simulink model "switching_deadtime_motor_model"  (R2023b)
settings: Solver=FixedStepDiscrete  StartTime=0.0  StopTime=0.002  FixedStep=ss_cfg.model_fixed_step_s  RelTol=1e-3
values from neighbouring files (symbols this model uses):
  phase = mod(t / T_pwm, 1.0)    [plot_phase_a_deadtime_comparison.m]    (also in run_mcu_sampling_window_study.m; run_rl_sampling_impact_study.m; run_rotating_rl_sampling_study.m; run_triangle_carrier_study.m)
  ss_cfg = local_parse_inputs(ss_cfg, varargin{:})    [run_switching_deadtime_motor_smoke_test.m]
libraries: simulink x2, spsDCVoltageSourceLib x1, motor_control_lib x1, spsPermanentMagnetSynchronousMachineLib x1, spsUniversalBridgeLib x1, spspowerguiLib x1
settings Model: DataDictionary=motor_control_interface.sldd  Creator=user  LastModifiedBy=user

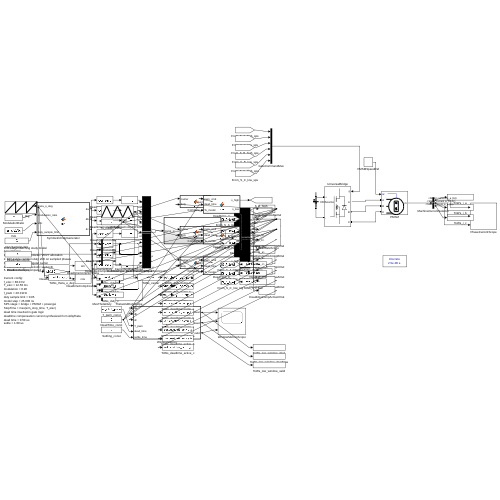
[thumbnail: Simulink's stored preview of the top-level diagram]
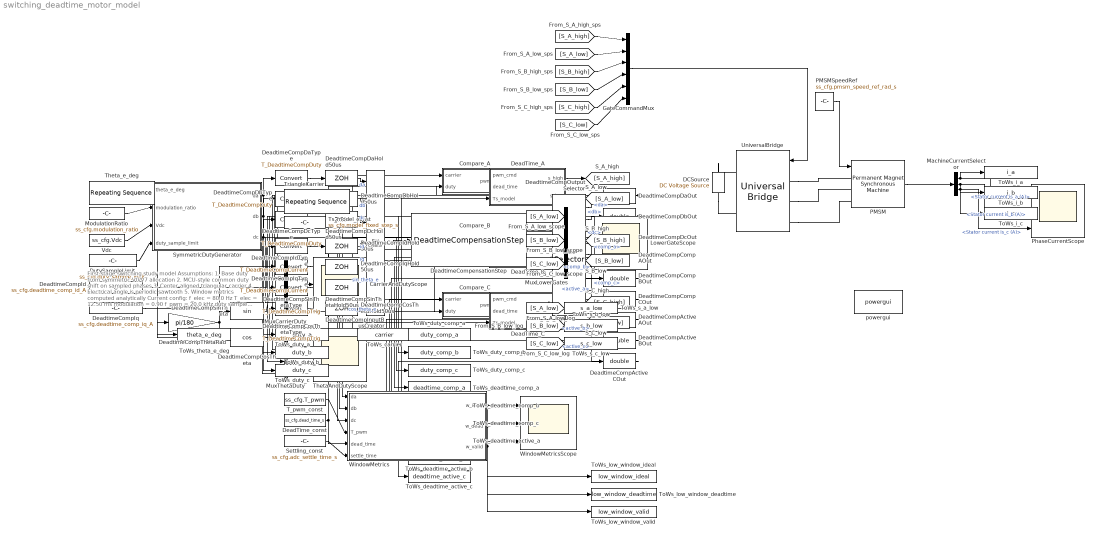
== system switching_deadtime_motor_model ==
  note: First-stage switching study model
      | Assumptions:
      | 1. Base duty from symmetric V0/V7 allocation
      | 2. MCU-style common duty shift on sampled phases
      | 3. Center-aligned triangular carrier
      | 4. Electrical angle is periodic sawtooth
      | 5. Window metrics computed analytically
      |
      | Current config:
      | f_elec = 80.0 Hz
      | T_elec = 12.50 ms
      | modulation = 0.90
      | f_pwm = 20.0 kHz
      | duty sample limit = 0.95
      | model step = 25.000 ns
      | SPS stage = bridge + PMSM + powergui
      | StopTime = max(sim_stop_time, T_elec)
      | dead time inserted in gate logic
      | deadtime compensation current synthesized from id/iq/theta
      | dead time = 0.50 us
      | settle = 1.00 us
  CarrierAndDutyScope : Scope
  Compare_A : MATLAB Function  TreatAsAtomicUnit=on
  Compare_B : MATLAB Function  TreatAsAtomicUnit=on
  Compare_C : MATLAB Function  TreatAsAtomicUnit=on
  DCSource : spsDCVoltageSourceLib/DC Voltage Source  Amplitude=ss_cfg.Vdc  Measurements=None
  DeadTime_A : MATLAB Function  TreatAsAtomicUnit=on
  DeadTime_B : MATLAB Function  TreatAsAtomicUnit=on
  DeadTime_C : MATLAB Function  TreatAsAtomicUnit=on
  DeadTime_const : Constant  Value=ss_cfg.dead_time_s
  DeadtimeCompActiveAOut : DataTypeConversion  OutDataTypeStr=double  SaturateOnIntegerOverflow=off  RndMeth=Floor
  DeadtimeCompActiveBOut : DataTypeConversion  OutDataTypeStr=double  SaturateOnIntegerOverflow=off  RndMeth=Floor
  DeadtimeCompActiveCOut : DataTypeConversion  OutDataTypeStr=double  SaturateOnIntegerOverflow=off  RndMeth=Floor
  DeadtimeCompCompAOut : DataTypeConversion  OutDataTypeStr=double  SaturateOnIntegerOverflow=off  RndMeth=Floor
  DeadtimeCompCompBOut : DataTypeConversion  OutDataTypeStr=double  SaturateOnIntegerOverflow=off  RndMeth=Floor
  DeadtimeCompCompCOut : DataTypeConversion  OutDataTypeStr=double  SaturateOnIntegerOverflow=off  RndMeth=Floor
  DeadtimeCompCosTheta : Trigonometry  Operator=cos
  DeadtimeCompCosThetaHold50us : ZeroOrderHold  SampleTime=ss_cfg.deadtime_comp_update_s
  DeadtimeCompCosThetaType : DataTypeConversion  OutDataTypeStr=T_DeadtimeCompTrig  SaturateOnIntegerOverflow=off  RndMeth=Floor
  DeadtimeCompDaHold50us : ZeroOrderHold  SampleTime=ss_cfg.deadtime_comp_update_s
  DeadtimeCompDaOut : DataTypeConversion  OutDataTypeStr=double  SaturateOnIntegerOverflow=off  RndMeth=Floor
  DeadtimeCompDaType : DataTypeConversion  OutDataTypeStr=T_DeadtimeCompDuty  SaturateOnIntegerOverflow=off  RndMeth=Floor
  DeadtimeCompDbHold50us : ZeroOrderHold  SampleTime=ss_cfg.deadtime_comp_update_s
  DeadtimeCompDbOut : DataTypeConversion  OutDataTypeStr=double  SaturateOnIntegerOverflow=off  RndMeth=Floor
  DeadtimeCompDbType : DataTypeConversion  OutDataTypeStr=T_DeadtimeCompDuty  SaturateOnIntegerOverflow=off  RndMeth=Floor
  DeadtimeCompDcHold50us : ZeroOrderHold  SampleTime=ss_cfg.deadtime_comp_update_s
  DeadtimeCompDcOut : DataTypeConversion  OutDataTypeStr=double  SaturateOnIntegerOverflow=off  RndMeth=Floor
  DeadtimeCompDcType : DataTypeConversion  OutDataTypeStr=T_DeadtimeCompDuty  SaturateOnIntegerOverflow=off  RndMeth=Floor
  DeadtimeCompId : Constant  Value=ss_cfg.deadtime_comp_id_A
  DeadtimeCompIdHold50us : ZeroOrderHold  SampleTime=ss_cfg.deadtime_comp_update_s
  DeadtimeCompIdType : DataTypeConversion  OutDataTypeStr=T_DeadtimeCompCurrent  SaturateOnIntegerOverflow=off  RndMeth=Floor
  DeadtimeCompInputBusCreator : BusCreator  Inputs=7  OutDataTypeStr=Bus: pwm_deadtime_comp_input_t  NonVirtualBus=on
  DeadtimeCompIq : Constant  Value=ss_cfg.deadtime_comp_iq_A
  DeadtimeCompIqHold50us : ZeroOrderHold  SampleTime=ss_cfg.deadtime_comp_update_s
  DeadtimeCompIqType : DataTypeConversion  OutDataTypeStr=T_DeadtimeCompCurrent  SaturateOnIntegerOverflow=off  RndMeth=Floor
  DeadtimeCompOutputSelector : BusSelector  OutputSignals=da,db,dc,comp_a,comp_b,comp_c,active_a,active_b,active_c
  DeadtimeCompSinTheta : Trigonometry
  DeadtimeCompSinThetaHold50us : ZeroOrderHold  SampleTime=ss_cfg.deadtime_comp_update_s
  DeadtimeCompSinThetaType : DataTypeConversion  OutDataTypeStr=T_DeadtimeCompTrig  SaturateOnIntegerOverflow=off  RndMeth=Floor
  DeadtimeCompThetaRad : Gain  Gain=pi/180
  DeadtimeCompensationStep : motor_control_lib/DeadtimeCompensationStep  SystemSampleTime=-1  VariantActivationTime=update diagram  AllowFlexibleInterface=on  Latency=0  AutoFrameSizeCalculation=off
      settings: SourceProductName=Motor Control Modules
  DutySampleLimit : Constant  Value=ss_cfg.duty_sample_limit
  GateCommandMux : Mux  Inputs=6
  LowerGateScope : Scope
  MachineCurrentSelector : BusSelector  OutputSignals=Stator current is_a (A),Stator current is_b (A),Stator current is_c (A)
  ModulationRatio : Constant  Value=ss_cfg.modulation_ratio
  MuxCarrierDuty : Mux
  MuxLowerGates : Mux  Inputs=3
  MuxThetaDuty : Mux
  PMSM : spsPermanentMagnetSynchronousMachineLib/Permanent Magnet Synchronous Machine  NbPhases=3  FluxDistribution=Sinusoidal  RotorType=Round  MechanicalLoad=Speed w  PresetModel=No  ShowDetailedParameters=on  MeasurementBus=off  Resistance=ss_cfg.pmsm_resistance_ohm  Inductance=ss_cfg.pmsm_inductance_h  dqInductances=[ss_cfg.pmsm_inductance_h, ss_cfg.pmsm_inductance_h]  La=0.000395  MachineConstant=Flux linkage established by magnets (V.s)  Flux=ss_cfg.pmsm_flux_wb  VoltageCst=13.0594  TorqueCst=0.108  Flat=120  Mechanical=ss_cfg.pmsm_mechanical  PolePairs=ss_cfg.pmsm_pole_pairs  InitialConditions=ss_cfg.pmsm_initial_conditions  InitialConditions5ph=[0 0 0 0 0 0]  RefAngle=90 degrees behind phase A axis (modified Park)  IterativeDiscreteModel=Trapezoidal non iterative  TsBlock=-1  TsPowergui=ss_cfg.powergui_sample_time_s
  PMSMSpeedRef : Constant  Value=ss_cfg.pmsm_speed_ref_rad_s
  PhaseCurrentScope : Scope  NumInputPorts=3
  Settling_const : Constant  Value=ss_cfg.adc_settle_time_s
  SymmetricDutyGenerator : MATLAB Function  TreatAsAtomicUnit=on
  T_pwm_const : Constant  Value=ss_cfg.T_pwm
  ThetaAndDutyScope : Scope
  Theta_e_deg : simulink/Sources/Repeating Sequence  rep_seq_t=[0 1/ss_cfg.electrical_freq_hz]  rep_seq_y=[0 360]
  ToWs_carrier : ToWorkspace  VariableName=carrier  SaveFormat=Structure With Time  SampleTime=-1
  ToWs_deadtime_active_a : ToWorkspace  VariableName=deadtime_active_a  SaveFormat=Structure With Time  SampleTime=-1
  ToWs_deadtime_active_b : ToWorkspace  VariableName=deadtime_active_b  SaveFormat=Structure With Time  SampleTime=-1
  ToWs_deadtime_active_c : ToWorkspace  VariableName=deadtime_active_c  SaveFormat=Structure With Time  SampleTime=-1
  ToWs_deadtime_comp_a : ToWorkspace  VariableName=deadtime_comp_a  SaveFormat=Structure With Time  SampleTime=-1
  ToWs_deadtime_comp_b : ToWorkspace  VariableName=deadtime_comp_b  SaveFormat=Structure With Time  SampleTime=-1
  ToWs_deadtime_comp_c : ToWorkspace  VariableName=deadtime_comp_c  SaveFormat=Structure With Time  SampleTime=-1
  ToWs_duty_a : ToWorkspace  VariableName=duty_a  SaveFormat=Structure With Time  SampleTime=-1
  ToWs_duty_b : ToWorkspace  VariableName=duty_b  SaveFormat=Structure With Time  SampleTime=-1
  ToWs_duty_c : ToWorkspace  VariableName=duty_c  SaveFormat=Structure With Time  SampleTime=-1
  ToWs_duty_comp_a : ToWorkspace  VariableName=duty_comp_a  SaveFormat=Structure With Time  SampleTime=-1
  ToWs_duty_comp_b : ToWorkspace  VariableName=duty_comp_b  SaveFormat=Structure With Time  SampleTime=-1
  ToWs_duty_comp_c : ToWorkspace  VariableName=duty_comp_c  SaveFormat=Structure With Time  SampleTime=-1
  ToWs_i_a : ToWorkspace  VariableName=i_a  SaveFormat=Structure With Time  SampleTime=-1
  ToWs_i_b : ToWorkspace  VariableName=i_b  SaveFormat=Structure With Time  SampleTime=-1
  ToWs_i_c : ToWorkspace  VariableName=i_c  SaveFormat=Structure With Time  SampleTime=-1
  ToWs_low_window_deadtime : ToWorkspace  VariableName=low_window_deadtime  SaveFormat=Structure With Time  SampleTime=-1
  ToWs_low_window_ideal : ToWorkspace  VariableName=low_window_ideal  SaveFormat=Structure With Time  SampleTime=-1
  ToWs_low_window_valid : ToWorkspace  VariableName=low_window_valid  SaveFormat=Structure With Time  SampleTime=-1
  ToWs_s_a_low : ToWorkspace  VariableName=s_a_low  SaveFormat=Structure With Time  SampleTime=-1
  ToWs_s_b_low : ToWorkspace  VariableName=s_b_low  SaveFormat=Structure With Time  SampleTime=-1
  ToWs_s_c_low : ToWorkspace  VariableName=s_c_low  SaveFormat=Structure With Time  SampleTime=-1
  ToWs_theta_e_deg : ToWorkspace  VariableName=theta_e_deg  SaveFormat=Structure With Time  SampleTime=-1
  TriangleCarrier : simulink/Sources/Repeating Sequence  rep_seq_t=[0 ss_cfg.T_pwm/2 ss_cfg.T_pwm]  rep_seq_y=[0 1 0]
  Ts_model_const : Constant  Value=ss_cfg.model_fixed_step_s
  UniversalBridge : spsUniversalBridgeLib/Universal Bridge  Arms=3  SnubberResistance=1e5  SnubberCapacitance=inf  Device=MOSFET / Diodes  Ron=1e-3  Lon=0  ForwardVoltages="[  0  0  ]"  ForwardVoltage=0  GTOparameters=[ 10e-6 , 20e-6 ]  IGBTparameters=[ 1e-6 , 2e-6 ]  Measurements=None  Measurements_2=None  converterType=Rectifier
  Vdc : Constant  Value=ss_cfg.Vdc
  WindowMetrics : MATLAB Function  TreatAsAtomicUnit=on
  WindowMetricsScope : Scope  NumInputPorts=3
  powergui : spspowerguiLib/powergui  Priority=1  SimulationMode=Discrete  SampleTime=ss_cfg.powergui_sample_time_s  frequency=60  Iterations=50  frequencyindice=60  Pbase=100e6  ErrMax=1e-4  UnitsV=kV  UnitsW=MW  buscounter=0  FunctionMessages=off  echomessages=off  EnableUseOfTLC=off  CurrentSourceSwitches=off  DisableSnubberDevices=off  DisableRonSwitches=off  DisableVfSwitches=off  DisplayEquations=off  AutomaticDiscreteSolvers=off  SolverType=Tustin/Backward Euler (TBE)  Interpol=off  ExternalGateDelay=off  methode=off  Ts=100  x0status=blocks  SPID=on  SwTol=0  HookPort=off  NonlinearTolerance=1e-4  nMaxIteration=100  ContinueOnMaxIteration=off  RestoreLinks=warning  ResistiveCurrentMeasurement=off  Frange=[0:2:500]  Ylog=off  Xlog=on  ShowGrid=off  save=off  variable=ZData  structure=0  ZoomFFT=off  StartTime=0.0  cycles=1  DisplayStyle=1  fundamental=60  FreqAxis=off  MaxFrequency=1000  frequencyindicesteady=1  RmsSteady=1  display=off
  wires:
  Theta_e_deg/1 -> SymmetricDutyGenerator/1(theta_e_deg), DeadtimeCompThetaRad/1, MuxThetaDuty/1, ToWs_theta_e_deg/1
  ModulationRatio/1 -> SymmetricDutyGenerator/2(modulation_ratio)
  Vdc/1 -> SymmetricDutyGenerator/3(Vdc)
  DutySampleLimit/1 -> SymmetricDutyGenerator/4(duty_sample_limit)
  DeadtimeCompThetaRad/1 -> DeadtimeCompSinTheta/1, DeadtimeCompCosTheta/1
  SymmetricDutyGenerator/1(da) -> DeadtimeCompDaType/1, ToWs_duty_a/1
  DeadtimeCompDaType/1 -> DeadtimeCompDaHold50us/1
  SymmetricDutyGenerator/2(db) -> DeadtimeCompDbType/1, ToWs_duty_b/1
  DeadtimeCompDbType/1 -> DeadtimeCompDbHold50us/1
  SymmetricDutyGenerator/3(dc) -> DeadtimeCompDcType/1, ToWs_duty_c/1
  DeadtimeCompDcType/1 -> DeadtimeCompDcHold50us/1
  DeadtimeCompId/1 -> DeadtimeCompIdType/1
  DeadtimeCompIdType/1 -> DeadtimeCompIdHold50us/1
  DeadtimeCompIq/1 -> DeadtimeCompIqType/1
  DeadtimeCompIqType/1 -> DeadtimeCompIqHold50us/1
  DeadtimeCompSinTheta/1 -> DeadtimeCompSinThetaType/1
  DeadtimeCompSinThetaType/1 -> DeadtimeCompSinThetaHold50us/1
  DeadtimeCompCosTheta/1 -> DeadtimeCompCosThetaType/1
  DeadtimeCompCosThetaType/1 -> DeadtimeCompCosThetaHold50us/1
  DeadtimeCompDaHold50us/1 -> DeadtimeCompInputBusCreator/1  "da"
  DeadtimeCompDbHold50us/1 -> DeadtimeCompInputBusCreator/2  "db"
  DeadtimeCompDcHold50us/1 -> DeadtimeCompInputBusCreator/3  "dc"
  DeadtimeCompIdHold50us/1 -> DeadtimeCompInputBusCreator/4  "id"
  DeadtimeCompIqHold50us/1 -> DeadtimeCompInputBusCreator/5  "iq"
  DeadtimeCompSinThetaHold50us/1 -> DeadtimeCompInputBusCreator/6  "sin_theta_e"
  DeadtimeCompCosThetaHold50us/1 -> DeadtimeCompInputBusCreator/7  "cos_theta_e"
  DeadtimeCompInputBusCreator/1 -> DeadtimeCompensationStep/1
  DeadtimeCompensationStep/1 -> DeadtimeCompOutputSelector/1
  DeadtimeCompOutputSelector/1 -> DeadtimeCompDaOut/1  "<da>"
  DeadtimeCompOutputSelector/2 -> DeadtimeCompDbOut/1  "<db>"
  DeadtimeCompOutputSelector/3 -> DeadtimeCompDcOut/1  "<dc>"
  DeadtimeCompOutputSelector/4 -> DeadtimeCompCompAOut/1  "<comp_a>"
  DeadtimeCompOutputSelector/5 -> DeadtimeCompCompBOut/1  "<comp_b>"
  DeadtimeCompOutputSelector/6 -> DeadtimeCompCompCOut/1  "<comp_c>"
  DeadtimeCompOutputSelector/7 -> DeadtimeCompActiveAOut/1  "<active_a>"
  DeadtimeCompOutputSelector/8 -> DeadtimeCompActiveBOut/1  "<active_b>"
  DeadtimeCompOutputSelector/9 -> DeadtimeCompActiveCOut/1  "<active_c>"
  TriangleCarrier/1 -> Compare_A/1(carrier), Compare_B/1(carrier), Compare_C/1(carrier), MuxCarrierDuty/1, ToWs_carrier/1
  DeadtimeCompDaOut/1 -> Compare_A/2(duty), MuxCarrierDuty/2, MuxThetaDuty/2, WindowMetrics/1(da), ToWs_duty_comp_a/1
  Compare_A/1(pwm_cmd) -> DeadTime_A/1(pwm_cmd)
  DeadTime_const/1 -> DeadTime_A/2(dead_time), DeadTime_B/2(dead_time), DeadTime_C/2(dead_time), WindowMetrics/5(dead_time)
  Ts_model_const/1 -> DeadTime_A/3(Ts_model), DeadTime_B/3(Ts_model), DeadTime_C/3(Ts_model)
  DeadTime_A/1(s_high) -> [S_A_high]
  DeadTime_A/2(s_low) -> [S_A_low]
  DeadtimeCompDbOut/1 -> Compare_B/2(duty), MuxCarrierDuty/3, MuxThetaDuty/3, WindowMetrics/2(db), ToWs_duty_comp_b/1
  Compare_B/1(pwm_cmd) -> DeadTime_B/1(pwm_cmd)
  DeadTime_B/1(s_high) -> [S_B_high]
  DeadTime_B/2(s_low) -> [S_B_low]
  DeadtimeCompDcOut/1 -> Compare_C/2(duty), MuxCarrierDuty/4, MuxThetaDuty/4, WindowMetrics/3(dc), ToWs_duty_comp_c/1
  Compare_C/1(pwm_cmd) -> DeadTime_C/1(pwm_cmd)
  DeadTime_C/1(s_high) -> [S_C_high]
  DeadTime_C/2(s_low) -> [S_C_low]
  MuxCarrierDuty/1 -> CarrierAndDutyScope/1
  MuxThetaDuty/1 -> ThetaAndDutyScope/1
  [S_A_low] -> MuxLowerGates/1
  [S_B_low] -> MuxLowerGates/2
  [S_C_low] -> MuxLowerGates/3
  MuxLowerGates/1 -> LowerGateScope/1
  [S_A_high] -> GateCommandMux/1
  [S_A_low] -> GateCommandMux/2
  [S_B_high] -> GateCommandMux/3
  [S_B_low] -> GateCommandMux/4
  [S_C_high] -> GateCommandMux/5
  [S_C_low] -> GateCommandMux/6
  GateCommandMux/1 -> UniversalBridge/1
  PMSMSpeedRef/1 -> PMSM/1
  PMSM/1 -> MachineCurrentSelector/1
  MachineCurrentSelector/1 -> PhaseCurrentScope/1, ToWs_i_a/1  "<Stator current is_a (A)>"
  MachineCurrentSelector/2 -> PhaseCurrentScope/2, ToWs_i_b/1  "<Stator current is_b (A)>"
  MachineCurrentSelector/3 -> PhaseCurrentScope/3, ToWs_i_c/1  "<Stator current is_c (A)>"
  T_pwm_const/1 -> WindowMetrics/4(T_pwm)
  Settling_const/1 -> WindowMetrics/6(settle_time)
  WindowMetrics/1(w_ideal) -> WindowMetricsScope/1, ToWs_low_window_ideal/1
  WindowMetrics/2(w_dead) -> WindowMetricsScope/2, ToWs_low_window_deadtime/1
  WindowMetrics/3(w_valid) -> WindowMetricsScope/3, ToWs_low_window_valid/1
  DeadtimeCompCompAOut/1 -> ToWs_deadtime_comp_a/1
  DeadtimeCompCompBOut/1 -> ToWs_deadtime_comp_b/1
  DeadtimeCompCompCOut/1 -> ToWs_deadtime_comp_c/1
  DeadtimeCompActiveAOut/1 -> ToWs_deadtime_active_a/1
  DeadtimeCompActiveBOut/1 -> ToWs_deadtime_active_b/1
  DeadtimeCompActiveCOut/1 -> ToWs_deadtime_active_c/1
  [S_A_low] -> ToWs_s_a_low/1
  [S_B_low] -> ToWs_s_b_low/1
  [S_C_low] -> ToWs_s_c_low/1
  connections:
  UniversalBridge/LConn1 -- PMSM/LConn1
  UniversalBridge/LConn2 -- PMSM/LConn2
  UniversalBridge/LConn3 -- PMSM/LConn3
  DCSource/RConn1 -- UniversalBridge/RConn1
  DCSource/LConn1 -- UniversalBridge/RConn2

== matlab function switching_deadtime_motor_model/Compare_A ==
  data: carrier input; pwm_cmd output; duty input
function pwm_cmd = fcn(carrier, duty)
% Boundary-safe PWM compare for duty in [0, 1]
if duty <= 0.0
    pwm_cmd = false;
elseif duty >= 1.0
    pwm_cmd = true;
else
    pwm_cmd = carrier < duty;
end
end

== matlab function switching_deadtime_motor_model/SymmetricDutyGenerator ==
  data: theta_e_deg input; da output; modulation_ratio input; Vdc input; duty_sample_limit input; db output; dc output
function [da, db, dc] = fcn(theta_e_deg, modulation_ratio, Vdc, duty_sample_limit)
% Symmetric V0/V7 base duty plus MCU-style common duty shift
theta_e = theta_e_deg * pi / 180;
v_mag = modulation_ratio * (Vdc / sqrt(3));
v_alpha = -v_mag * sin(theta_e);
v_beta =  v_mag * cos(theta_e);
va = v_alpha;
vb = -0.5 * v_alpha + sqrt(3) / 2 * v_beta;
vc = -0.5 * v_alpha - sqrt(3) / 2 * v_beta;
duty_raw = [va; vb; vc] / Vdc + 0.5;
shift_min = -min(duty_raw);
shift_max = 1.0 - max(duty_raw);
shift = 0.5 * (shift_min + shift_max);
duty = min(max(duty_raw + shift, 0.0), 1.0);
if (va >= vb) && (vb >= vc)
    sector = 1;
elseif (vb >= va) && (va >= vc)
    sector = 2;
elseif (vb >= vc) && (vc >= va)
    sector = 3;
elseif (vc >= vb) && (vb >= va)
    sector = 4;
elseif (vc >= va) && (va >= vb)
    sector = 5;
else
    sector = 6;
end
duty_a = duty(1);
duty_b = duty(2);
duty_c = duty(3);
switch sector
    case {1, 6}
        max_sampled = max(duty_b, duty_c);
    case {2, 3}
        max_sampled = max(duty_a, duty_c);
    case {4, 5}
        max_sampled = max(duty_a, duty_b);
    otherwise
        max_sampled = 0.0;
end
if max_sampled > duty_sample_limit
    common_shift = -(max_sampled - duty_sample_limit);
    min_duty = min([duty_a; duty_b; duty_c]);
    if (min_duty + common_shift) < 0.0
        common_shift = -min_duty;
    end
    duty_a = duty_a + common_shift;
    duty_b = duty_b + common_shift;
    duty_c = duty_c + common_shift;
end
duty = min(max([duty_a; duty_b; duty_c], 0.0), 1.0);
da = duty(1);
db = duty(2);
dc = duty(3);
end

== matlab function switching_deadtime_motor_model/DeadTime_A ==
  data: pwm_cmd input; s_high output; dead_time input; Ts_model input; s_low output
function [s_high, s_low] = fcn(pwm_cmd, dead_time, Ts_model)
% Complementary gate generation with dead time
persistent active_state pending_state dead_count initialized
if isempty(initialized)
    active_state = double(pwm_cmd >= 0.5);
    pending_state = active_state;
    dead_count = 0;
    initialized = true;
end
requested_state = double(pwm_cmd >= 0.5);
samples_dt = max(1, ceil(dead_time / Ts_model));
if dead_time <= 0.0
    active_state = requested_state;
    dead_count = 0;
elseif dead_count > 0
    pending_state = requested_state;
    dead_count = dead_count - 1;
    if dead_count == 0
        active_state = pending_state;
    else
        active_state = -1;
    end
elseif requested_state ~= active_state
    pending_state = requested_state;
    active_state = -1;
    dead_count = samples_dt;
end
if active_state == 1
    s_high = true;
    s_low = false;
elseif active_state == 0
    s_high = false;
    s_low = true;
else
    s_high = false;
    s_low = false;
end
end

== matlab function switching_deadtime_motor_model/Compare_B ==
  data: carrier input; pwm_cmd output; duty input
function pwm_cmd = fcn(carrier, duty)
% Boundary-safe PWM compare for duty in [0, 1]
if duty <= 0.0
    pwm_cmd = false;
elseif duty >= 1.0
    pwm_cmd = true;
else
    pwm_cmd = carrier < duty;
end
end

== matlab function switching_deadtime_motor_model/DeadTime_B ==
  data: pwm_cmd input; s_high output; dead_time input; Ts_model input; s_low output
function [s_high, s_low] = fcn(pwm_cmd, dead_time, Ts_model)
% Complementary gate generation with dead time
persistent active_state pending_state dead_count initialized
if isempty(initialized)
    active_state = double(pwm_cmd >= 0.5);
    pending_state = active_state;
    dead_count = 0;
    initialized = true;
end
requested_state = double(pwm_cmd >= 0.5);
samples_dt = max(1, ceil(dead_time / Ts_model));
if dead_time <= 0.0
    active_state = requested_state;
    dead_count = 0;
elseif dead_count > 0
    pending_state = requested_state;
    dead_count = dead_count - 1;
    if dead_count == 0
        active_state = pending_state;
    else
        active_state = -1;
    end
elseif requested_state ~= active_state
    pending_state = requested_state;
    active_state = -1;
    dead_count = samples_dt;
end
if active_state == 1
    s_high = true;
    s_low = false;
elseif active_state == 0
    s_high = false;
    s_low = true;
else
    s_high = false;
    s_low = false;
end
end

== matlab function switching_deadtime_motor_model/Compare_C ==
  data: carrier input; pwm_cmd output; duty input
function pwm_cmd = fcn(carrier, duty)
% Boundary-safe PWM compare for duty in [0, 1]
if duty <= 0.0
    pwm_cmd = false;
elseif duty >= 1.0
    pwm_cmd = true;
else
    pwm_cmd = carrier < duty;
end
end

== matlab function switching_deadtime_motor_model/DeadTime_C ==
  data: pwm_cmd input; s_high output; dead_time input; Ts_model input; s_low output
function [s_high, s_low] = fcn(pwm_cmd, dead_time, Ts_model)
% Complementary gate generation with dead time
persistent active_state pending_state dead_count initialized
if isempty(initialized)
    active_state = double(pwm_cmd >= 0.5);
    pending_state = active_state;
    dead_count = 0;
    initialized = true;
end
requested_state = double(pwm_cmd >= 0.5);
samples_dt = max(1, ceil(dead_time / Ts_model));
if dead_time <= 0.0
    active_state = requested_state;
    dead_count = 0;
elseif dead_count > 0
    pending_state = requested_state;
    dead_count = dead_count - 1;
    if dead_count == 0
        active_state = pending_state;
    else
        active_state = -1;
    end
elseif requested_state ~= active_state
    pending_state = requested_state;
    active_state = -1;
    dead_count = samples_dt;
end
if active_state == 1
    s_high = true;
    s_low = false;
elseif active_state == 0
    s_high = false;
    s_low = true;
else
    s_high = false;
    s_low = false;
end
end

== matlab function switching_deadtime_motor_model/WindowMetrics ==
  data: da input; w_ideal output; db input; dc input; T_pwm input; dead_time input; settle_time input; w_dead output; w_valid output
function [w_ideal, w_dead, w_valid] = fcn(da, db, dc, T_pwm, dead_time, settle_time)
% Low-side window metrics for center-aligned PWM
d = [da; db; dc];
w_ideal = zeros(3,1);
w_dead = zeros(3,1);
w_valid = zeros(3,1);
for i = 1:3
    w_ideal(i) = max((1.0 - d(i)) * T_pwm, 0.0);
    w_dead(i) = max(w_ideal(i) - 2.0 * dead_time, 0.0);
    w_valid(i) = max(w_dead(i) - settle_time, 0.0);
end
end
